simulink model "last_successful"  (R2023a)
settings: Solver=VariableStepAuto  StartTime=0.0  StopTime=inf  RelTol=1e-3
model workspace (MAT data in the model file):
  Rtot = 1.2947
undefined symbols (not defined in the file): CR, LF
libraries: instrumentseriallib x2
settings Model: Creator=husey  LastModifiedBy=husey

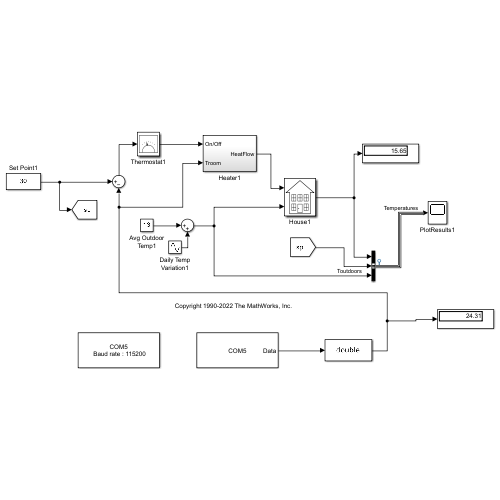
[thumbnail: Simulink's stored preview of the top-level diagram]
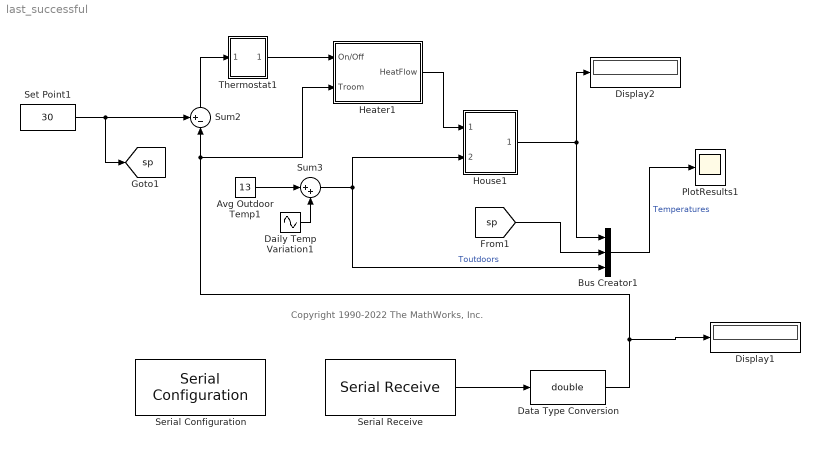
== system last_successful ==
  note: Copyright 1990-2022 The MathWorks, Inc.
  Avg Outdoor Temp1 : Constant  Value=13
  Bus Creator1 : BusCreator  Inputs=3
  Daily Temp Variation1 : Sin  Amplitude=15  Frequency=1/2400  SampleTime=0
  Data Type Conversion : DataTypeConversion  OutDataTypeStr=double  SaturateOnIntegerOverflow=off  RndMeth=Floor
  Display1 : Display
  Display2 : Display
  Heater1 : Subsystem
  House1 : Subsystem
      mask Display: image('HouseHeatHousePix.svg'); % Use "Edit Image" on toolstrip to change.
  PlotResults1 : Scope
  Serial Configuration : instrumentseriallib/Serial Configuration  Priority=-200000  PortSel=COM5  Port=COM5  ComPort=COM5  BaudRate=115200  DataBits=8  Parity=none  StopBits=1  ByteOrder=little-endian  FlowControl=none  Timeout=10  SimulateUsing=Interpreted execution  BlockInModel=on  aMode=1
  Serial Receive : instrumentseriallib/Serial Receive  Priority=1  PortSel=COM5  Port=COM5  ComPort=COM5  DataType=single  SaveDataType=uint8  ToggleHeader=off  Header=[]  ToggleTerminator=off  Terminator=CR/LF ('\r\n')  CustomTerminator=[]  InputFormat=Row major  ToggleDataSize=on  DataSize=[1 1]  EnableBlockingMode=on  ActionDataUnavailable=Output last received value  ActionWhenDataUnavailable=Output last received value  CustomValue=0  SampleTime=1  SimulateUsing=Interpreted execution  BlockInModel=on  aMode=1
  Set Point1 : Constant  Value=30
  Sum2 : Sum  Inputs=+-|  InputSameDT=on  SaturateOnIntegerOverflow=on  OutDataTypeStr=Inherit: Same as first input
  Sum3 : Sum  Inputs=|++  InputSameDT=on  SaturateOnIntegerOverflow=on  OutDataTypeStr=Inherit: Same as first input
  Thermostat1 : Subsystem
      mask Display: image('HouseHeatThermostatPix.svg'); % Use "Edit Image" on toolstrip to change.
  tag scope: sp=global
  wires:
  Sum3/1 -> House1/2(Outdoor Temp Tout1), Bus Creator1/3  "Toutdoors"
  Heater1/1(HeatFlow) -> House1/1(Tinitial)
  Serial Receive/1 -> Data Type Conversion/1
  Bus Creator1/1 -> PlotResults1/1  "Temperatures"
  Avg Outdoor Temp1/1 -> Sum3/1
  House1/1(Room Temp Troom1) -> Display2/1, Bus Creator1/1
  Sum2/1 -> Thermostat1/1(Terr)
  Data Type Conversion/1 -> Display1/1, Heater1/2(Troom), Sum2/2
  Set Point1/1 -> Sum2/1, [sp]
  Daily Temp Variation1/1 -> Sum3/2
  [sp] -> Bus Creator1/2
  Thermostat1/1(Blower switch) -> Heater1/1(On/Off)

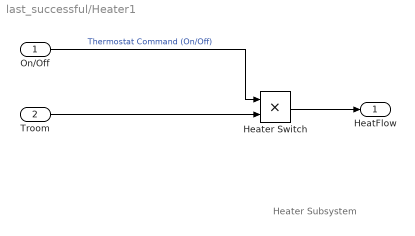
== system last_successful/Heater1 ==
  note: Heater Subsystem
  On/Off : Inport  SampleTime=1
  Troom : Inport  Port=2
  Heater Switch : Product  OutDataTypeStr=Inherit: Keep MSB  RndMeth=Nearest
  HeatFlow : Outport  VectorParamsAs1DForOutWhenUnconnected=off
  wires:
  On/Off/1 -> Heater Switch/1  "Thermostat Command (On/Off)"
  Troom/1 -> Heater Switch/2
  Heater Switch/1 -> HeatFlow/1

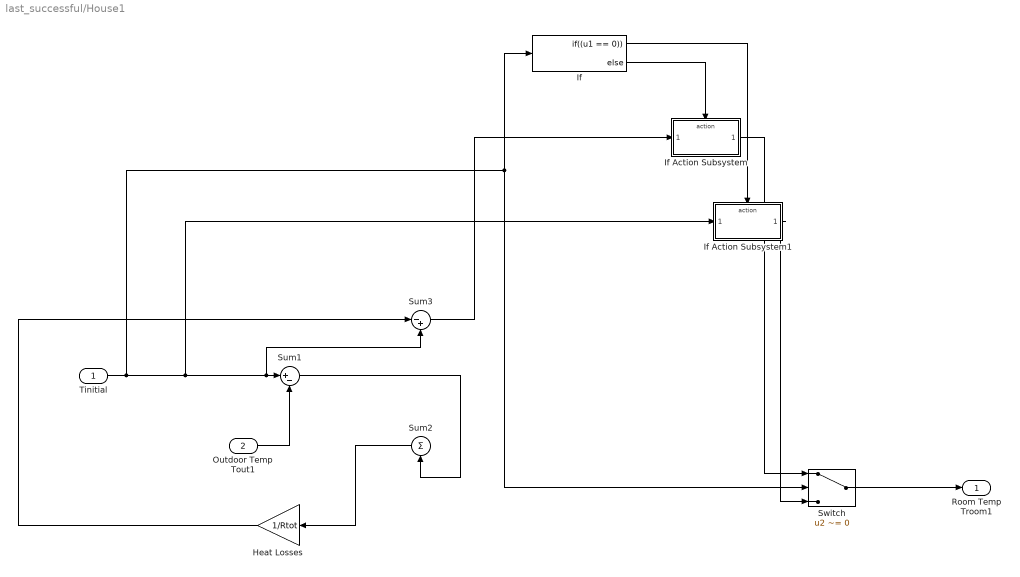
== system last_successful/House1 ==
  Tinitial : Inport
  Outdoor Temp Tout1 : Inport  Port=2
  Heat Losses : Gain  Gain=1/Rtot  SaturateOnIntegerOverflow=on  OutDataTypeStr=Inherit: Same as input  ParamDataTypeStr=Inherit: Same as input
  If : If  IfExpression=(u1 == 0)  ZeroCross=off
  If Action Subsystem : Subsystem  TreatAsAtomicUnit=on
  If Action Subsystem1 : Subsystem  TreatAsAtomicUnit=on
  Sum1 : Sum  Inputs=|+-  InputSameDT=on  SaturateOnIntegerOverflow=on  OutDataTypeStr=Inherit: Same as first input
  Sum2 : Sum  Inputs=|+  InputSameDT=on  SaturateOnIntegerOverflow=on  OutDataTypeStr=Inherit: Same as first input
  Sum3 : Sum  Inputs=|-+  InputSameDT=on  SaturateOnIntegerOverflow=on  OutDataTypeStr=Inherit: Same as first input
  Switch : Switch  Criteria=u2 ~= 0  SaturateOnIntegerOverflow=off  InputSameDT=off
  Room Temp Troom1 : Outport  InitialOutput=0  VectorParamsAs1DForOutWhenUnconnected=off
  wires:
  Tinitial/1 -> If Action Subsystem1/1(HeatFlow), Sum1/1, Sum3/2, Switch/2, If/1
  Sum1/1 -> Sum2/1
  Sum2/1 -> Heat Losses/1
  Outdoor Temp Tout1/1 -> Sum1/2
  Heat Losses/1 -> Sum3/1
  If/2 -> If Action Subsystem/Action
  If/1 -> If Action Subsystem1/Action
  If Action Subsystem/1(Room Temp Troom1) -> Switch/1
  If Action Subsystem1/1(Room Temp Troom2) -> Switch/3
  Sum3/1 -> If Action Subsystem/1(HeatFlow)
  Switch/1 -> Room Temp Troom1/1

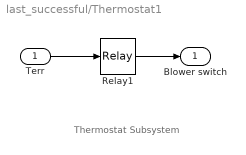
== system last_successful/Thermostat1 ==
  note: Thermostat Subsystem
  Terr : Inport
  Relay1 : Relay  OnSwitchValue=5*(5/9)  OffSwitchValue=-5*(5/9)
  Blower switch : Outport  InitialOutput=0  VectorParamsAs1DForOutWhenUnconnected=off
  wires:
  Terr/1 -> Relay1/1
  Relay1/1 -> Blower switch/1

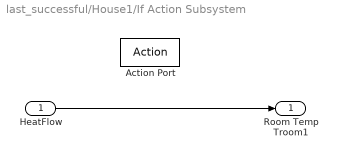
== system last_successful/House1/If Action Subsystem ==
  HeatFlow : Inport
  Action Port : ActionPort  ActionPortLabel=else
  Room Temp Troom1 : Outport
  wires:
  HeatFlow/1 -> Room Temp Troom1/1

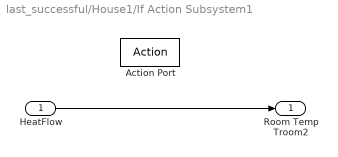
== system last_successful/House1/If Action Subsystem1 ==
  HeatFlow : Inport
  Action Port : ActionPort  ActionPortLabel=if((u1 == 0))
  Room Temp Troom2 : Outport
  wires:
  HeatFlow/1 -> Room Temp Troom2/1
